simulink model "NRZ_PROJECT"  (R2024b)
settings: Solver=ode23tb  StartTime=0.0  StopTime=50  RelTol=1e-3
libraries: simulink_extras x5, spspowerguiLib x1
settings Model: Creator=Ayush kumar das  LastModifiedBy=Ayush kumar das

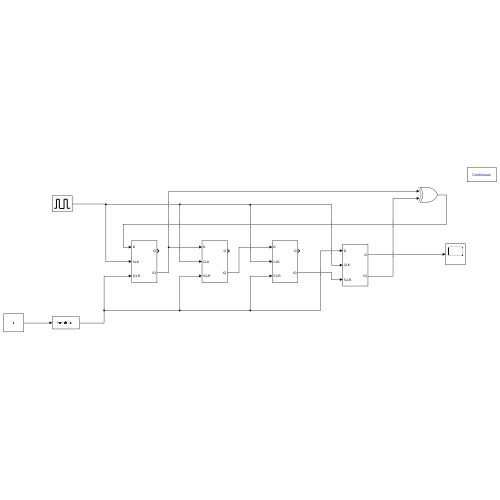
[thumbnail: Simulink's stored preview of the top-level diagram]
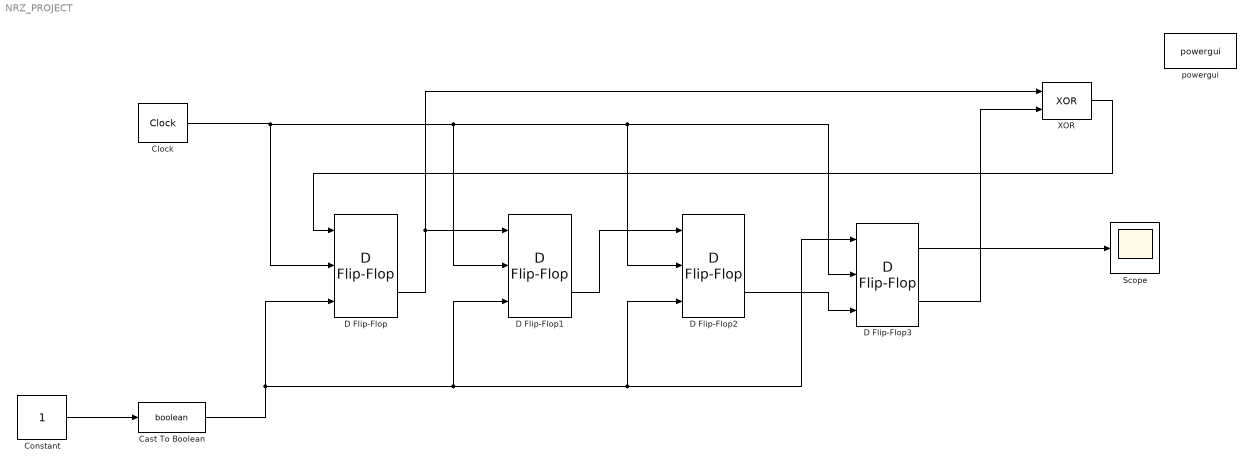
== system NRZ_PROJECT ==
  Cast To Boolean : DataTypeConversion  OutDataTypeStr=boolean  SaturateOnIntegerOverflow=off  RndMeth=Floor
  Clock : simulink_extras/Flip Flops/Clock  period=2
  Constant : Constant
  D Flip-Flop{,1..3} (4 alike) : simulink_extras/Flip Flops/D Flip-Flop
  Scope : Scope
  XOR : Logic  Operator=XOR  IconShape=distinctive  AllPortsSameDT=off  OutDataTypeStr=boolean
  powergui : spspowerguiLib/powergui  Priority=1  SimulationMode=Continuous  SampleTime=50e-6  frequency=60  Iterations=50  frequencyindice=60  Pbase=100e6  ErrMax=1e-4  UnitsV=kV  UnitsW=MW  buscounter=0  FunctionMessages=off  echomessages=off  EnableUseOfTLC=off  CurrentSourceSwitches=off  DisableSnubberDevices=off  DisableRonSwitches=off  DisableVfSwitches=off  DisplayEquations=off  AutomaticDiscreteSolvers=off  SolverType=Tustin/Backward Euler (TBE)  Interpol=off  ExternalGateDelay=off  methode=off  Ts=100  x0status=blocks  SPID=on  SwTol=0  HookPort=off  NonlinearTolerance=1e-4  nMaxIteration=100  ContinueOnMaxIteration=off  RestoreLinks=warning  ResistiveCurrentMeasurement=off  Frange=[0:2:500]  Ylog=off  Xlog=on  ShowGrid=off  save=off  variable=ZData  structure=0  ZoomFFT=off  StartTime=0.0  cycles=1  DisplayStyle=1  fundamental=60  FreqAxis=off  MaxFrequency=1000  frequencyindicesteady=1  RmsSteady=1  display=off
  wires:
  Clock/1 -> D Flip-Flop3/2, D Flip-Flop2/2, D Flip-Flop1/2, D Flip-Flop/2
  Constant/1 -> Cast To Boolean/1
  XOR/1 -> D Flip-Flop/1
  D Flip-Flop/2 -> D Flip-Flop1/1, XOR/1
  D Flip-Flop3/2 -> XOR/2
  D Flip-Flop2/2 -> D Flip-Flop3/3
  D Flip-Flop1/2 -> D Flip-Flop2/1
  D Flip-Flop3/1 -> Scope/1
  Cast To Boolean/1 -> D Flip-Flop1/3, D Flip-Flop2/3, D Flip-Flop3/1, D Flip-Flop/3
